simulink model "SEL751_Test_F2"  (Simulink 8.1)
settings: Solver=ode4  StartTime=0.0  StopTime=inf  FixedStep=Ts  MaxStep=1e-3  RelTol=1e-3
model workspace (MAT data in the model file):
  op_snapshot1 : opcond.OperatingPoint (value not decoded)
PostLoadFcn:
  | Ts=100e-6; HILLTOP_init;SIM_HIL=1
InitFcn:
  | Ts=100e-6; HILLTOP_init;SIM_HIL=1
undefined symbols (not defined in the file or in its folder): EX, FF, OP5142_1
libraries: rtio_opalrt_common x4, rtlab x2, cables_lib x2, breaker_lib x2, powerlib x2, Load_lib x2, artemis x1, simulink_extras x1, transformer_lib x1
settings Model: ARTEMISmethode_block_infos=$$__separator__$$SEL751_Test_F2/ARTEMIS Guide$$__separator__$$  Creator=RE25624  LastModifiedBy=ed12083  BufferReuse=off
settings SolverCC: ZeroCrossAlgorithm=Adaptive
settings DataIOCC: ExternalInput=getinputstruct(op_snapshot1)  InitialState=getstatestruct(op_snapshot1)  LimitDataPoints=off  MaxDataPoints=90060  SignalLoggingSaveFormat=Dataset  SaveOutput=off  SignalLogging=off  DSMLogging=off  SaveTime=off  OutputSaveName=result
settings OptimizationCC: BlockReduction=off  OptimizeBlockIOStorage=off  BufferReuse=off  ExpressionFolding=off  LocalBlockOutputs=off
settings DebuggingCC: MaxConsecutiveZCsMsg=warning  IgnoredZcDiagnostic=none  SolverPrmCheckMsg=none  MultiTaskRateTransMsg=warning  FcnCallInpInsideContextMsg=EnableAllAsWarning  FrameProcessingCompatibilityMsg=error  ModelReferenceExtraNoncontSigs=warning  StrictBusMsg=None
settings ModelReferenceCC: UpdateModelReferenceTargets=IfOutOfDate
settings SFSimCC: SFSimEcho=off
settings GRTTargetCC: CodeReplacementLibrary=C89/C90 (ANSI)

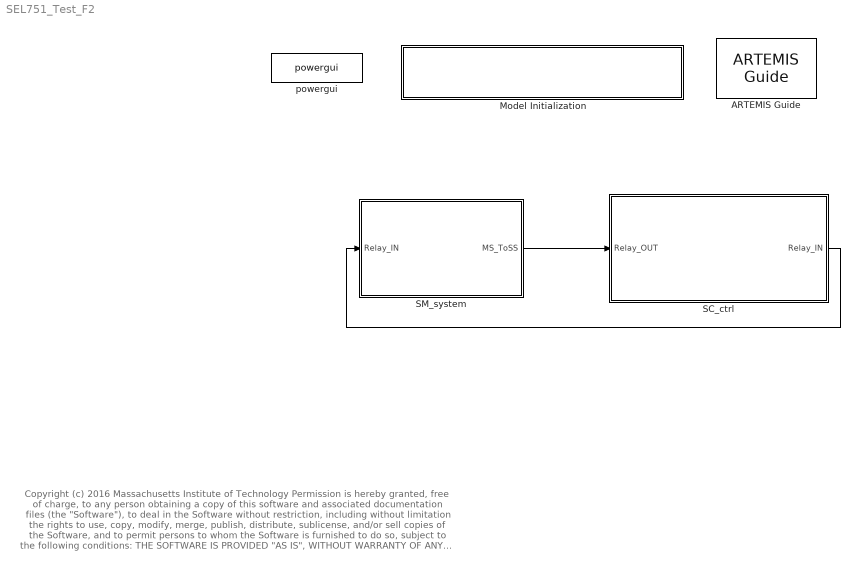
== system SEL751_Test_F2 ==
  note: Copyright (c) 2016 Massachusetts Institute of Technology
      | Permission is hereby granted, free of charge, to any person obtaining a copy of this software and associated documentation files (the "Software"), to deal
      | in the Software without restriction, including without limitation the rights to use, copy, modify, merge, publish, distribute, sublicense, and/or sell copies of the
      | Software, and to permit persons to whom the Software is furnished to do so, subject to the following conditions:
      |
      | THE SOFTWARE IS PROVIDED "AS IS", WITHOUT WARRANTY OF ANY KIND, EXPRESS OR IMPLIED, INCLUDING BUT NOT LIMITED TO THE
      | WARRANTIES OF MERCHANTABILITY, FITNESS FOR A PARTICULAR PURPOSE AND NONINFRINGEMENT. IN NO EVENT SHALL THE AUTHORS
      | OR COPYRIGHT HOLDERS BE LIABLE FOR ANY CLAIM, DAMAGES OR OTHER LIABILITY, WHETHER IN AN ACTION OF CONTRACT, TORT OR
      | OTHERWISE, ARISING FROM, OUT OF OR IN CONNECTION WITH THE SOFTWARE OR THE USE OR OTHER DEALINGS IN THE SOFTWARE.
  ARTEMIS Guide : artemis/ARTEMIS/ARTEMIS Guide  Tag=FTSSmethode_opal_4hx0r99  Description=5.0_z1  lock=on  Ts=Ts  opt=art5  dyna=off  nb_perm=4  RT_fullcomp=off  ssn=on  ssn_itvc=off  ssn_ivic=off  ssn_ext=off  ssn_solver=Art5 with Backward Euler nodal interface  ssn_impulse=off  ssn_quasimpulse=off  ssn_impulse_loop=2  paraExtinctionThy=off  Thy_Impulse=on  dtc=Off  dtc_opt=normal  ao=on  simtype=off  ct_mac=off  lin_mov=off  lsp=[0.001 2]  spike_skip=Disabled  dtc_extra=1  dtc_sws=normal  dtc_pied=0.5  SPSRulesBlock=SPSRules  tre=on  ctmm=off  LF=off  dpl_type=ARTEMiS DPL  rlc_type=off  custom_type=off  para=on  ssn_ImpulseLoopBlockedStateUpdate=2  ssn_mov_iter_number=5  ssn_switch_iter_number=5
  Model Initialization : Subsystem  AncestorBlock=artemis/Tools /Misc/Model Initialization  mask(Model Functions){InitFcnX=Ts=100e-6; HILLTOP_init;SIM_HIL=1, prel=off, posl=on, inif=on, strf=off}
      mask prompts: InitFcnX "Initialisation"; prel "Preload Function"; posl "PostLoad Function"; inif "InitFcn"; strf "StartFcn"
      mask init:
      | currentBlock = gcb;
      | root = bdroot(currentBlock);
      | 
      | 
      | if ~strcmp(get_param(root,'BlockDiagramType'),'library')
      |     if prel==1
      |         set_param(root, 'PreLoadFcn', InitFcnX);
      |     else
      |         set_param(root, 'PreLoadFcn', '');
      |     end
      |     if inif==1
      |         set_param(root, 'InitFcn', InitFcnX);
      |     else
      |         set_param(root, 'InitFcn', '');
      |     end
      |     if strf==1
      |         set_param(root, 'StartFcn', InitFcnX);
      |     else
      |         set_param(root, 'StartFcn', '');
      |     end
      |     if posl==1
      |         set_param(root, 'PostLoadFcn', InitFcnX);
      |     else
      |         set_param(root, 'PostLoadFcn', '');
      |     end
      | end
      | 
      | pos = get_param(currentBlock, 'Position');
      | width = pos(3) - pos(1); height = pos(4) - pos(2);
      | txt = [ upper(root) '\n' '- InitFcn. . . . . '  get_param(root, 'InitFcn') ];
      settings: CopyFcn=set_param(gcb,'LinkStatus','inactive')
      mask Display: text(5, height*0.5, txt, 'horizontalAlignment', 'left', 'verticalAlignment', 'middle') ;
  SC_ctrl : Subsystem
  SM_system : Subsystem
  powergui : powerlib/powergui  Priority=2  SimulationMode=Discrete  SolverType=Tustin  SampleTime=Ts  frequency=60  SPID=off  DisableSnubberDevices=off  DisableRonSwitches=off  DisableVfSwitches=off  SwTol=0  Interpol=off  DisplayEquations=off  frequencyindice=0  Pbase=100e6  ErrMax=1e-4  Iterations=50  UnitsV=kV  UnitsW=MW  FunctionMessages=off  echomessages=off  HookPort=off  EnableUseOfTLC=off  x0status=blocks  RestoreLinks=warning  ResistiveCurrentMeasurement=off  Frange=logspace(0,3,50)  Ylog=off  Xlog=off  ShowGrid=off  save=off  variable=ZData  structure=0  ZoomFFT=on  StartTime=0.0  cycles=2  DisplayStyle=off  fundamental=60  FreqAxis=off  MaxFrequency=1000  frequencyindicesteady=1  RmsSteady=1  display=off  Ts=0  methode=off
  wires:
  SM_system/1(MS_ToSS) -> SC_ctrl/1(Relay_OUT)
  SC_ctrl/1(Relay_IN) -> SM_system/1(Relay_IN)

== system SEL751_Test_F2/Model Initialization ==

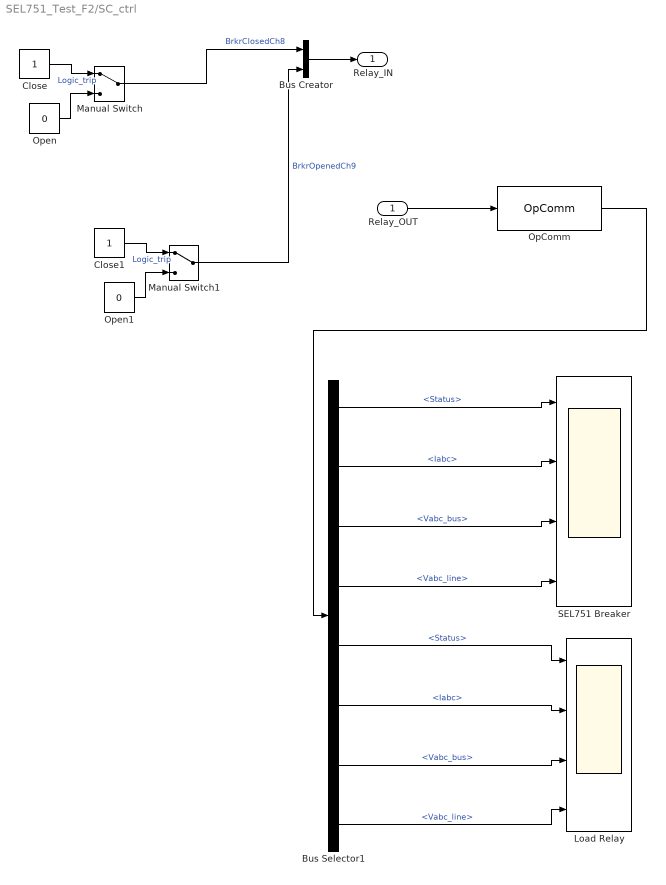
== system SEL751_Test_F2/SC_ctrl ==
  Relay_OUT : Inport
  Bus Creator : BusCreator  Inputs=2
  Bus Selector1 : BusSelector  OutputSignals=SEL751_1.Status,SEL751_1.Iabc,SEL751_1.Vabc_bus,SEL751_1.Vabc_line,relay_2.Status,relay_2.Iabc,relay_2.Vabc_bus,relay_2.Vabc_line
  Close : Constant
  Close1 : Constant
  Load Relay : Scope  NumInputPorts=4
      settings: TimeRange=1  YMin=0.95~-200~-400~-400  YMax=1.05~200~400~400  SaveName=ScopeData4
  Manual Switch : ManualSwitch
  Manual Switch1 : ManualSwitch
  OpComm : rtlab/OpComm  nbport=1  groupe_acq=1  subsys_rate=0  st=0  Synchronization=on  Interpolation=on  Threshold=1.0  Missed_Data=off  Sim_Time=off  Samples=off  dynSigOut=off  from_console=0  warning_done=off  writeOpCommFile=off  Offset=off
  Open : Constant  Value=0
  Open1 : Constant  Value=0
  SEL751 Breaker : Scope  NumInputPorts=4
      settings: TimeRange=1  YMin=-1~-9~-70~-12500  YMax=1~8~80~12500  SaveName=ScopeData2
  Relay_IN : Outport
  wires:
  OpComm/1 -> Bus Selector1/1
  Relay_OUT/1 -> OpComm/1
  Close/1 -> Manual Switch/1  "Logic_trip"
  Open/1 -> Manual Switch/2
  Close1/1 -> Manual Switch1/1  "Logic_trip"
  Open1/1 -> Manual Switch1/2
  Bus Creator/1 -> Relay_IN/1
  Manual Switch1/1 -> Bus Creator/2  "BrkrOpenedCh9"
  Manual Switch/1 -> Bus Creator/1  "BrkrClosedCh8"
  Bus Selector1/1 -> SEL751 Breaker/1  "<Status>"
  Bus Selector1/2 -> SEL751 Breaker/2  "<Iabc>"
  Bus Selector1/3 -> SEL751 Breaker/3  "<Vabc_bus>"
  Bus Selector1/4 -> SEL751 Breaker/4  "<Vabc_line>"
  Bus Selector1/5 -> Load Relay/1  "<Status>"
  Bus Selector1/6 -> Load Relay/2  "<Iabc>"
  Bus Selector1/7 -> Load Relay/3  "<Vabc_bus>"
  Bus Selector1/8 -> Load Relay/4  "<Vabc_line>"

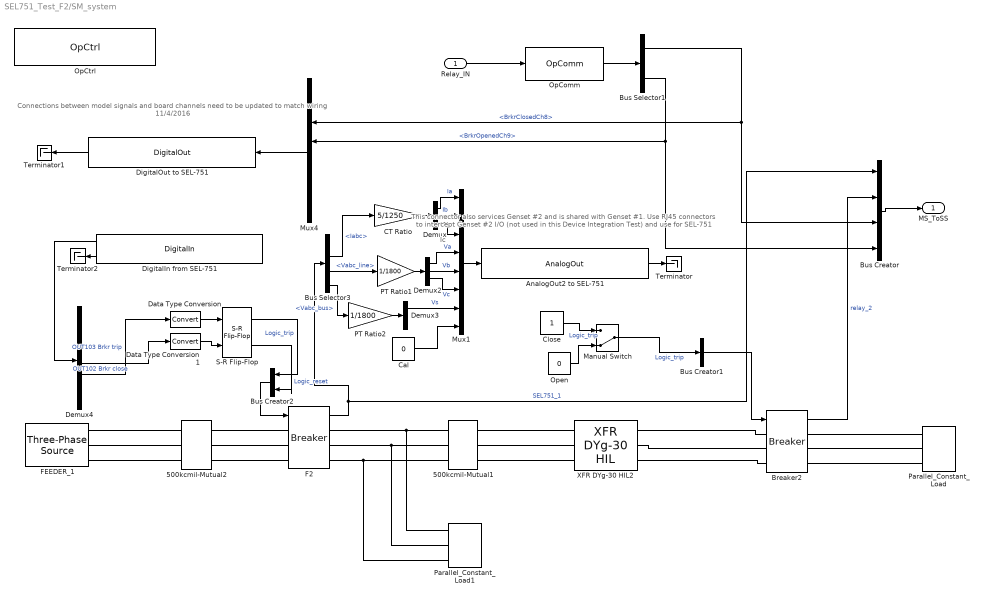
== system SEL751_Test_F2/SM_system ==
  note: This connector also services Genset #2 and  is
      | shared with Genset #1.  Use RJ45 connectors to
      |  intercept Genset #2 I/O (not used in this Device
      | Integration Test) and use for SEL-751
  note: Connections between model signals and board
      | channels need to be updated to match wiring
      | 11/4/2016
  note: Ic
  Relay_IN : Inport
  500kcmil-Mutual1 : cables_lib/500kcmil-Mutual  length=5000  par_sets=1  ratio=3
  500kcmil-Mutual2 : cables_lib/500kcmil-Mutual  length=5000  par_sets=1  ratio=3
  AnalogOut2 to SEL-751 : rtio_opalrt_common/AnalogOut  CtrlName='OpCtrl'  portNb=2  FcnNos=Slot 1 Module A Subsection 2  size=16  maxcount=8  count=8  numchan=8  israngeinput=off  voltagerange=[ -5 ... 5 ]  slot=0  side=0  mismatch=0  slotside=Slot_1_Module_A
      settings: AttributesFormatString=%<CtrlName>
  Breaker2 : breaker_lib/Breaker  Ts=Ts  mech_delay=cb_mech_delay
  Bus Creator : BusCreator
  Bus Creator1 : BusCreator  Inputs=1
  Bus Creator2 : BusCreator  Inputs=2
  Bus Selector1 : BusSelector  OutputSignals=BrkrClosedCh8,BrkrOpenedCh9
  Bus Selector3 : BusSelector  OutputSignals=Status,Iabc,Vabc_line,Vabc_bus
  CT Ratio : Gain  Gain=5/1250
  Cal : Constant  Value=0
  Close : Constant
  Data Type Conversion : DataTypeConversion
  Data Type Conversion1 : DataTypeConversion
  Demux : Demux  Outputs=3
  Demux2 : Demux  Outputs=3
  Demux3 : Demux  Outputs=3
  Demux4 : Demux  Outputs=8
  DigitalIn from SEL-751 : rtio_opalrt_common/DigitalIn  CtrlName='OpCtrl'  portNb=3  FcnNos=Slot 4 Module A Subsection 1  size=1  maxcount=8  count=8  sampleTime=0  numchan=8
      settings: AttributesFormatString=%<CtrlName>
  DigitalOut to SEL-751 : rtio_opalrt_common/DigitalOut  CtrlName='OpCtrl'  portNb=9  FcnNos=Slot 3 Module B Subsection 1  size=1  maxcount=8  count=8  numchan=8
      settings: AttributesFormatString=%<CtrlName>
  F2 : breaker_lib/Breaker  Ts=Ts  mech_delay=cb_mech_delay
  FEEDER_1 : powerlib/Electrical Sources/Three-Phase Source  Voltage=13800  PhaseAngle=0  Frequency=60  InternalConnection=Yg  SpecifyImpedance=on  Resistance=0.8929  Inductance=16.58e-3  ShortCircuitLevel=375e6  BaseVoltage=13800  XRratio=7.9  BusType=swing  Pref=0  Qref=0  Qmin=-inf  Qmax=inf
  Manual Switch : ManualSwitch  CurrentSetting=0
  Mux1 : Mux  Inputs=8
  Mux4 : Mux  Inputs=8
  OpComm : rtlab/OpComm  nbport=1  groupe_acq=1  subsys_rate=0  st=0  Synchronization=on  Interpolation=on  Threshold=1.0  Missed_Data=off  Sim_Time=off  Samples=off  dynSigOut=off  from_console=1  warning_done=off  writeOpCommFile=off  Offset=off
  OpCtrl : rtio_opalrt_common/OpCtrl  CtrlName='OpCtrl'  boardid=1  BitstreamFilename=OP5142_1-EX-0000-2_3_4_54-16AIO_48AO_32DO_16DIO_16selDIO_CD-FF-01  numconfig=-1  mode=Master  externalClock=off  decimRtsi=0  calibIO=off  SampleTime=0  loadinport=-1  BoardType=OP5142  SecondaryPresent=off  sync_type=Audio
  Open : Constant  Value=0
  PT Ratio1 : Gain  Gain=1/1800
  PT Ratio2 : Gain  Gain=1/1800
  Parallel_Constant_Load : Load_lib/Parallel_Constant_Load  v=460  kVA=100  pf=0.90
  Parallel_Constant_Load1 : Load_lib/Parallel_Constant_Load  v=13800  kVA=10000  pf=1
  S-R Flip-Flop : simulink_extras/Flip Flops/S-R Flip-Flop  initial_condition=1
  Terminator : Terminator
  Terminator1 : Terminator
  Terminator2 : Terminator
  XFR DYg-30 HIL2 : transformer_lib/XFR DYg-30 HIL  Rating=2500  Vp=13800  Vs=460  Z=5.18  XR=2.5
  MS_ToSS : Outport
  wires:
  Bus Creator/1 -> MS_ToSS/1
  Bus Creator1/1 -> Breaker2/1
  Mux1/1 -> AnalogOut2 to SEL-751/1
  Bus Selector3/2 -> CT Ratio/1  "<Iabc>"
  Demux/1 -> Mux1/1  "Ia"
  Demux/2 -> Mux1/2  "Ib"
  Demux/3 -> Mux1/3
  Demux2/1 -> Mux1/4  "Va"
  Demux2/2 -> Mux1/5  "Vb"
  Bus Selector3/4 -> PT Ratio2/1  "<Vabc_bus>"
  Demux3/1 -> Mux1/7  "Vs"
  Bus Selector3/3 -> PT Ratio1/1  "<Vabc_line>"
  Cal/1 -> Mux1/8
  AnalogOut2 to SEL-751/1 -> Terminator/1
  DigitalIn from SEL-751/1 -> Demux4/1
  Demux4/6 -> Data Type Conversion/1  "OUT103 Brkr trip"
  Data Type Conversion/1 -> S-R Flip-Flop/1
  Data Type Conversion1/1 -> S-R Flip-Flop/2
  S-R Flip-Flop/1 -> Bus Creator2/1  "Logic_trip"
  S-R Flip-Flop/2 -> Bus Creator2/2  "Logic_reset"
  Bus Creator2/1 -> F2/1
  Mux4/1 -> DigitalOut to SEL-751/1
  DigitalOut to SEL-751/1 -> Terminator1/1
  DigitalIn from SEL-751/2 -> Terminator2/1
  Breaker2/1 -> Bus Creator/2  "relay_2"
  F2/1 -> Bus Creator/1, Bus Selector3/1  "SEL751_1"
  Manual Switch/1 -> Bus Creator1/1  "Logic_trip"
  Close/1 -> Manual Switch/1  "Logic_trip"
  Open/1 -> Manual Switch/2
  CT Ratio/1 -> Demux/1
  PT Ratio1/1 -> Demux2/1
  PT Ratio2/1 -> Demux3/1
  Demux4/5 -> Data Type Conversion1/1  "OUT102 Brkr close"
  Relay_IN/1 -> OpComm/1
  OpComm/1 -> Bus Selector1/1
  Bus Selector1/1 -> Mux4/3, Bus Creator/3  "<BrkrClosedCh8>"
  Bus Selector1/2 -> Mux4/4, Bus Creator/4  "<BrkrOpenedCh9>"
  Demux2/3 -> Mux1/6  "Vc"
  connections:
  500kcmil-Mutual2/LConn2 -- FEEDER_1/RConn2
  500kcmil-Mutual2/LConn1 -- FEEDER_1/RConn1
  500kcmil-Mutual2/LConn3 -- FEEDER_1/RConn3
  XFR DYg-30 HIL2/LConn1 -- 500kcmil-Mutual1/RConn1
  XFR DYg-30 HIL2/LConn2 -- 500kcmil-Mutual1/RConn2
  XFR DYg-30 HIL2/LConn3 -- 500kcmil-Mutual1/RConn3
  500kcmil-Mutual1/LConn1 -- Parallel_Constant_Load1/RConn1 -- F2/RConn1
  500kcmil-Mutual1/LConn2 -- Parallel_Constant_Load1/RConn2 -- F2/RConn2
  500kcmil-Mutual1/LConn3 -- Parallel_Constant_Load1/RConn3 -- F2/RConn3
  XFR DYg-30 HIL2/RConn3 -- Breaker2/LConn3
  XFR DYg-30 HIL2/RConn2 -- Breaker2/LConn2
  XFR DYg-30 HIL2/RConn1 -- Breaker2/LConn1
  500kcmil-Mutual2/RConn1 -- F2/LConn1
  500kcmil-Mutual2/RConn2 -- F2/LConn2
  500kcmil-Mutual2/RConn3 -- F2/LConn3
  Parallel_Constant_Load/RConn1 -- Breaker2/RConn1
  Parallel_Constant_Load/RConn2 -- Breaker2/RConn2
  Parallel_Constant_Load/RConn3 -- Breaker2/RConn3
